simulink model "Thermal_Home_Model"  (R2023b)
settings: Solver=VariableStepAuto  StartTime=0.0  StopTime=10.0  RelTol=1e-3
libraries: simulink_extras x2
settings Model: Creator=3.22  LastModifiedBy=3.22

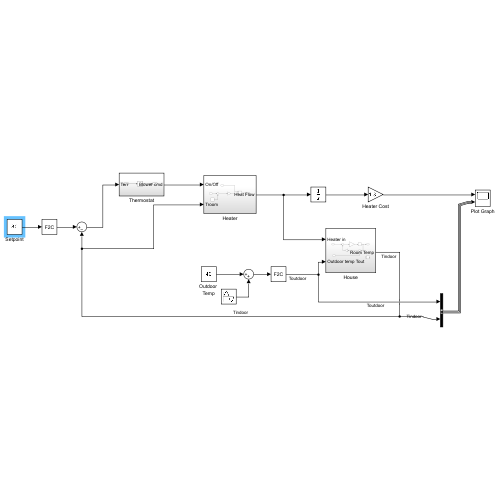
[thumbnail: Simulink's stored preview of the top-level diagram]
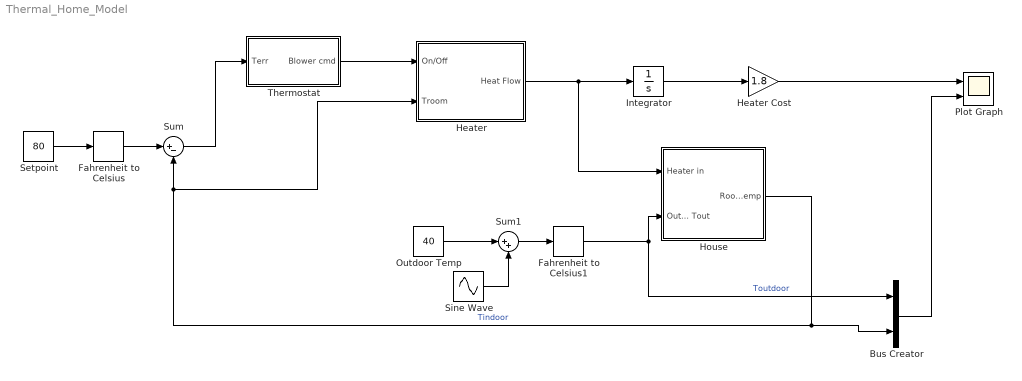
== system Thermal_Home_Model ==
  Bus Creator : BusCreator  Inputs=2
  Fahrenheit to Celsius : simulink_extras/Transformations/Fahrenheit to Celsius
  Fahrenheit to Celsius1 : simulink_extras/Transformations/Fahrenheit to Celsius
  Heater : Subsystem
  Heater Cost : Gain  Gain=1.8
  House : Subsystem
  Integrator : Integrator
  Outdoor Temp : Constant  Value=40
  Plot Graph : Scope  NumInputPorts=2
  Setpoint : Constant  Value=80
  Sine Wave : Sin  Amplitude=15  Frequency=2*pi/24  SampleTime=0
  Sum : Sum  Inputs=|+-
  Sum1 : Sum  Inputs=|++
  Thermostat : Subsystem
  wires:
  Sum/1 -> Thermostat/1(Terr)
  Setpoint/1 -> Fahrenheit to Celsius/1
  Fahrenheit to Celsius/1 -> Sum/1
  Fahrenheit to Celsius1/1 -> House/2(Outdoor temp Tout), Bus Creator/1  "Toutdoor"
  Thermostat/1(Blower cmd) -> Heater/1(On/Off)
  Heater/1(Heat Flow) -> Integrator/1, House/1(Heater in)
  House/1(Room Temp) -> Heater/2(Troom), Sum/2, Bus Creator/2  "Tindoor"
  Outdoor Temp/1 -> Sum1/1
  Sum1/1 -> Fahrenheit to Celsius1/1
  Sine Wave/1 -> Sum1/2
  Integrator/1 -> Heater Cost/1
  Heater Cost/1 -> Plot Graph/1
  Bus Creator/1 -> Plot Graph/2

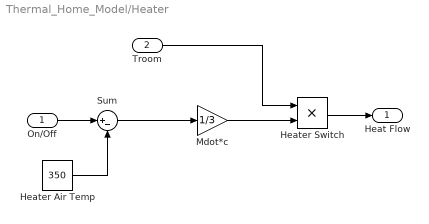
== system Thermal_Home_Model/Heater ==
  On/Off : Inport
  Troom : Inport  Port=2
  Heater Air Temp : Constant  Value=350
  Heater Switch : Product
  Mdot*c : Gain  Gain=1/3
  Sum : Sum  Inputs=|+-
  Heat Flow : Outport
  wires:
  On/Off/1 -> Sum/1
  Heater Switch/1 -> Heat Flow/1
  Sum/1 -> Mdot*c/1
  Mdot*c/1 -> Heater Switch/2
  Troom/1 -> Heater Switch/1
  Heater Air Temp/1 -> Sum/2

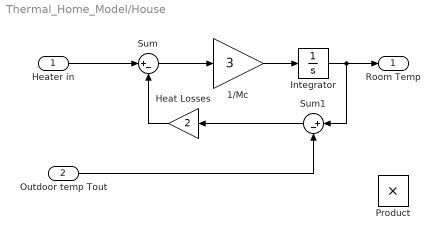
== system Thermal_Home_Model/House ==
  Heater in : Inport
  Outdoor temp Tout : Inport  Port=2
  1/Mc : Gain  Gain=3
  Heat Losses : Gain  Description=1/req  Gain=2
  Integrator : Integrator
  Product : Product
  Sum : Sum  Inputs=|+-
  Sum1 : Sum  Inputs=|+-
  Room Temp : Outport
  wires:
  1/Mc/1 -> Integrator/1
  Heater in/1 -> Sum/1
  Sum/1 -> 1/Mc/1
  Integrator/1 -> Sum1/1, Room Temp/1
  Sum1/1 -> Heat Losses/1
  Heat Losses/1 -> Sum/2
  Outdoor temp Tout/1 -> Sum1/2

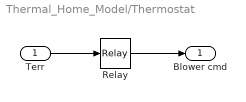
== system Thermal_Home_Model/Thermostat ==
  Terr : Inport
  Relay : Relay  OnSwitchValue=5*(5/9)  OffSwitchValue=-5*(5/9)
  Blower cmd : Outport
  wires:
  Relay/1 -> Blower cmd/1
  Terr/1 -> Relay/1
